simulink model "Particulas"  (R2020b)
settings: Solver=ode45  StartTime=0.0  StopTime=200  FixedStep=1e-7  RelTol=1e-4  AbsTol=1e-4  EnableMultiTasking=on
settings Model: EnablePacing=on  PacingRate=2  Creator=André  LastModifiedBy=Andre
settings SolverCC: AutoScaleAbsTol=off  ConsecutiveZCsStepRelTol=100*128*eps  ShapePreserveControl=EnableAll  ZeroCrossControl=EnableAll  AutoInsertRateTranBlk=on
settings DataIOCC: LimitDataPoints=on  SaveFormat=Array  SignalLoggingSaveFormat=ModelDataLogs  ReturnWorkspaceOutputs=off
settings OptimizationCC: ExpressionDepthLimit=2147483647  LifeSpan=inf
settings DebuggingCC: UnderspecifiedInitializationDetection=Classic  MergeDetectMultiDrivingBlocksExec=none  SolverPrmCheckMsg=warning  FcnCallInpInsideContextMsg=warning  StateNameClashWarn=warning  SFUnexpectedBacktrackingDiag=warning  SFNoUnconditionalDefaultTransitionDiag=warning  SFExecutionAtInitializationDiag=none  ArithmeticOperatorsInVariantConditions=warning
settings HardwareCC: ProdBitPerPointer=32  ProdBitPerSizeT=32  ProdBitPerPtrDiffT=32  ProdLargestAtomicFloat=None  ProdIntDivRoundTo=Undefined  ProdEndianess=Unspecified  ProdWordSize=32  ProdHWDeviceType=32-bit Generic
settings ModelReferenceCC: PropagateSignalLabelsOutOfModel=off
settings SFSimCC: SimUseLocalCustomCode=off  SimParseCustomCode=off  CustomCodeUndefinedFunction=UseInterfaceOnly
settings RTWCC: RTWUseLocalCustomCode=off
settings CodeAppCC: StateflowObjectComments=on
settings GRTTargetCC: TargetLangStandard=C89/C90 (ANSI)  CombineOutputUpdateFcns=off  GRTInterface=on
settings ConfigComp: CovMetricSettings=dw  CovSaveCumulativeToWorkspaceVar=on  CovSaveSingleToWorkspaceVar=on  CovExternalEMLEnable=off

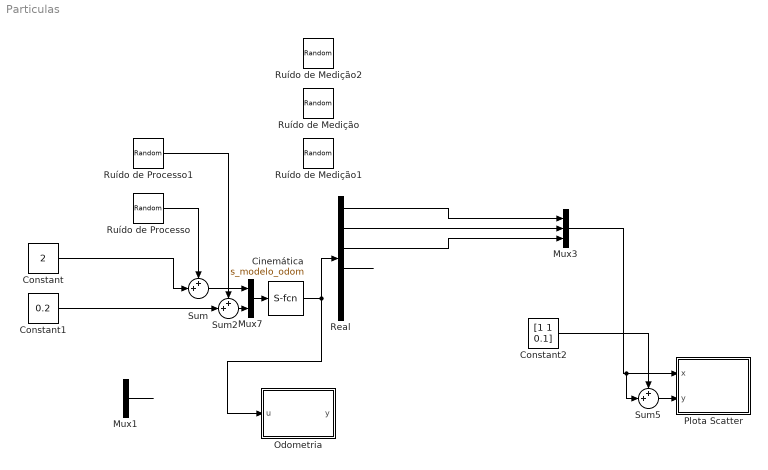
== system Particulas ==
  Cinemática : S-Function  FunctionName=s_modelo_odom  Parameters=[1 -5 0]  SFunctionDeploymentMode=off  EnableBusSupport=off
  Constant : Constant  Value=2
  Constant1 : Constant  Value=0.2
  Constant2 : Constant  Value=[1 1 0.1]
  Mux1 : Mux  Inputs=2
  Mux3 : Mux  Inputs=3
  Mux7 : Mux  Inputs=2
  Odometria : MATLAB Function  TreatAsAtomicUnit=on
  Plota Scatter : MATLAB Function  TreatAsAtomicUnit=on
  Real : Demux  Outputs=6
  Ruído de Medição : RandomNumber  Variance=0.1  SampleTime=0.01
  Ruído de Medição1 : RandomNumber  Variance=0.1  SampleTime=0.01
  Ruído de Medição2 : RandomNumber  Variance=0.1  SampleTime=0.01
  Ruído de Processo : RandomNumber  Variance=0.1  SampleTime=0.1
  Ruído de Processo1 : RandomNumber  Variance=0.1  SampleTime=0.1
  Sum : Sum  Inputs=++|
  Sum2 : Sum  Inputs=++|
  Sum5 : Sum  Inputs=++|
  wires:
  Mux1/1 -> ?
  Mux7/1 -> Cinemática/1
  Sum2/1 -> Mux7/2
  Constant/1 -> Sum/2
  Sum/1 -> Mux7/1
  Cinemática/1 -> Odometria/1(u), Real/1
  Constant1/1 -> Sum2/2
  Real/4 -> ?
  Real/1 -> Mux3/1
  Real/2 -> Mux3/2
  ? -> ?
  Ruído de Processo/1 -> Sum/1
  Mux3/1 -> Sum5/2, Plota Scatter/1(x)
  Ruído de Processo1/1 -> Sum2/1
  Real/3 -> Mux3/3
  Sum5/1 -> Plota Scatter/2(y)
  Constant2/1 -> Sum5/1

== matlab function Particulas/Odometria ==
  data: u input; y output
function y = fcn(u)
 
[x_ ,y_,th_,x_l,y_l,th_l] = u(:);

d_rot_1=atan2(y_l-y_,x_l,x_)-th_;
d_trans = sqrt((x_-x_l)^2 + (y_-y_l)^2);
d_rot_2 = th_l-th_-d_rot_1;





y = u;

== matlab function Particulas/Plota Scatter ==
  data: x input; y input
function  fcn(x,y)
     %n_Particulas = 1000;  
     %marker = [0 0; 5 5; 0 5]; % Positions of markers
     eixos =[-50 50 -50 50];
     %n_estados = n_Particulas*3;

     coder.extrinsic('scatter')
     coder.extrinsic('subplot')
     coder.extrinsic('quiver')
     coder.extrinsic('wrapToPi')
     subplot(1,1,1);
     % particulas = u(:);
     % xP = reshape(particulas,4,[]);
     % xP(3,:) = wrapToPi(xP(3,:) );
     % x_ = mean(xP(1:3,:).*([1 1 1]'*xP(4,:)), 2)/mean(xP(4,:));
     
     % scatter(xP(1,:),xP(2,:), 'k.');


      title('PF');
      scatter(y(1),y(2),'bo');
      hold on;
      quiver(y(1),y(2),cos(y(3)),sin(y(3)),5,'Color','b','LineWidth',0.5,'MaxHeadSize',0.6);
      
      
      axis( eixos);
      grid on;
      
      scatter(x(1),x(2), 'r*');
      quiver(x(1),x(2),cos(x(3)),sin(x(3)),5,'Color','r','LineWidth',0.5,'MaxHeadSize',0.4);
      hold off;
